simulink model "Target_Control_System"  (R2021b)
settings: Solver=FixedStepDiscrete  StartTime=0.0  StopTime=5  RelTol=1e-3
PreLoadFcn:
  | RTWConfigurationCB('preloadfcn', bdroot);
PostLoadFcn:
  | load('configuration/data_struct.mat');
  | load('configuration/fluxMaps_propMotor.mat');
  | load('configuration/parameterInit_PROP.mat');
  | load('configuration/parameterInit_PUMP.mat');
  | load('configuration/parameterInit_PITCH.mat');
  | load('configuration/parameterInit_TILT.mat');
  | %load('configuration/base_workspace_signal_definition.mat');
  | %load('resolvedatastores_to_baseworkspace_for_faster_simulation.mat');
model workspace (MAT data in the model file):
  SIMULATION_OPTIONS : Simulink.Parameter (value not decoded)
  TARGET_CODE_GEN : Simulink.Parameter (value not decoded)
  TCS_SAMPLE_FREQ_HZ : Simulink.Parameter (value not decoded)
symbols that are objects in the model workspace (value not decoded): TARGET_CODE_GEN, TCS_SAMPLE_FREQ_HZ
undefined symbols (not defined in the file): A_DQ_REF_LPF_INIT__PITCH, A_DQ_REF_LPF_INIT__PROP, A_DQ_REF_LPF_INIT__PUMP, A_DQ_REF_LPF_INIT__TILT, A_OBSERVER_CONFIDENCE_INIT__PITCH, A_OBSERVER_CONFIDENCE_INIT__PROP, A_OBSERVER_CONFIDENCE_INIT__PUMP, A_OBSERVER_CONFIDENCE_INIT__TILT, ACTUATOR_MAX_ANGLE_TRIP__PITCH, ACTUATOR_MIN_ANGLE_TRIP__PITCH, ACTUATOR_POS_SENSOR_INV_DIRECTION__PITCH, ACTUATOR_POS_SENSOR_INV_DIRECTION__TILT, ACTUATOR_POS_SENSOR_OFFSET__PITCH, ACTUATOR_POS_SENSOR_OFFSET__TILT, ADC_scaler1_baseaddr_TILT, ADC_SCALER_FLOAT_TO_FIXPOINT_EXPANSION, ANGLE_ELEC_FROM_SENSOR_OFFSET_INIT__PITCH, ANGLE_ELEC_FROM_SENSOR_OFFSET_INIT__PROP, ANGLE_ELEC_FROM_SENSOR_OFFSET_INIT__PUMP, ANGLE_ELEC_FROM_SENSOR_OFFSET_INIT__TILT, AUTO_CLEAR_FAULTS_ENABLED__PITCH, AUTO_CLEAR_FAULTS_ENABLED__PROP, AUTO_CLEAR_FAULTS_ENABLED__PUMP, AUTO_CLEAR_FAULTS_ENABLED__TILT, AUTO_CLEAR_FAULTS_WAIT_TICKS__PITCH, AUTO_CLEAR_FAULTS_WAIT_TICKS__PROP, AUTO_CLEAR_FAULTS_WAIT_TICKS__PUMP, AUTO_CLEAR_FAULTS_WAIT_TICKS__TILT, AUTO_I_ZERO_IDLE_TICKS__PITCH, AUTO_I_ZERO_IDLE_TICKS__PROP, AUTO_I_ZERO_IDLE_TICKS__PUMP, AUTO_I_ZERO_IDLE_TICKS__TILT, AUTO_I_ZERO_OFFSET_IDC_THRESHOLD__PITCH, AUTO_I_ZERO_OFFSET_IDC_THRESHOLD__PROP, AUTO_I_ZERO_OFFSET_IDC_THRESHOLD__PUMP, AUTO_I_ZERO_OFFSET_IDC_THRESHOLD__TILT, AUTO_I_ZERO_OFFSET_IPH_THRESHOLD__PITCH, AUTO_I_ZERO_OFFSET_IPH_THRESHOLD__PROP, AUTO_I_ZERO_OFFSET_IPH_THRESHOLD__PUMP, AUTO_I_ZERO_OFFSET_IPH_THRESHOLD__TILT, AUTO_SENSORLESS_SWITCHOVER_DISABLE_OMEGA, AUTO_SENSORLESS_SWITCHOVER_ENABLE_OMEGA, AUTO_SENSORLESS_SWITCHOVER_MIN_CONFIDENCE, AUXILIARY_PROTECTION_UNIT_BASEADDR__TILT, blanking_max_error_omega_INIT_PITCH, blanking_max_error_omega_INIT_TILT, blanking_max_error_position_INIT_PITCH, blanking_max_error_position_INIT_TILT, BRUTE_START_I_Q_REF_RAMP_SPEED__PITCH, BRUTE_START_I_Q_REF_RAMP_SPEED__PROP, BRUTE_START_I_Q_REF_RAMP_SPEED__PUMP, BRUTE_START_I_Q_REF_RAMP_SPEED__TILT, CONTROL_LOOP_DT_INIT__PITCH, CONTROL_LOOP_DT_INIT__PROP, CONTROL_LOOP_DT_INIT__PUMP, CONTROL_LOOP_DT_INIT__TILT, CORRECTION_FILTER_SCALE__PITCH, CORRECTION_FILTER_SCALE__PROP, CORRECTION_FILTER_SCALE__PUMP, CORRECTION_FILTER_SCALE__TILT ... (+458)
libraries: simulink x178, Reusables_Lib x24
(part 35 of 47)

== system Target_Control_System/Target_Control_System/MainLoop/tiltMotor_mainLoop/mainTask_tilt/motorTaskMainFastStep(&oTilt)/Control Loops - Tilt/Position Controller Tilt ==
  oRampDataPos_.fRampOut : Inport
  Enable : EnablePort
  Connect PosController to CurrentController : Subsystem
  Data Store Read1 : DataStoreRead  DataStoreName=oTilt  DataStoreElements=oTilt.oMot_.oParam_.fPosition2currentPMultiplier_  IndexOptions=Index vector (dialog)  Indices=1  OutputSizes=1
  Data Store Read10 : DataStoreRead  DataStoreName=oTilt  DataStoreElements=oTilt.oMot_.oState_.oPosSensor_.oPidDataPosCtrl_.oParameter_.ipInhibitTarget_  IndexOptions=Index vector (dialog)  Indices=1  OutputSizes=1
  Data Store Read11 : DataStoreRead  DataStoreName=oTilt  DataStoreElements=oTilt.oMot_.oState_.oPosSensor_.oPidDataPosCtrl_.oParameter_.fLoopDt_  IndexOptions=Index vector (dialog)  Indices=1  OutputSizes=1
  Data Store Read12 : DataStoreRead  DataStoreName=oTilt  DataStoreElements=oTilt.oMot_.oState_.oPosSensor_.oPidDataPosCtrl_.oParameter_.fIntMax_  IndexOptions=Index vector (dialog)  Indices=1  OutputSizes=1
  Data Store Read13 : DataStoreRead  DataStoreName=oTilt  DataStoreElements=oTilt.oMot_.oState_.oPosSensor_.oPidDataPosCtrl_.oParameter_.fIntMin_  IndexOptions=Index vector (dialog)  Indices=1  OutputSizes=1
  Data Store Read14 : DataStoreRead  DataStoreName=oTilt  DataStoreElements=oTilt.oMot_.oState_.oPosSensor_.oPidDataPosCtrl_.oParameter_.fIntegratorLeakFactor_  IndexOptions=Index vector (dialog)  Indices=1  OutputSizes=1
  Data Store Read15 : DataStoreRead  DataStoreName=oTilt  DataStoreElements=oTilt.oMot_.oState_.oPosSensor_.oPidDataPosCtrl_.oParameter_.fKd_  IndexOptions=Index vector (dialog)  Indices=1  OutputSizes=1
  Data Store Read16 : DataStoreRead  DataStoreName=oTilt  DataStoreElements=oTilt.oMot_.oState_.oPosSensor_.fOmegaEFromSensor_  IndexOptions=Index vector (dialog)  Indices=1  OutputSizes=1
  Data Store Read17 : DataStoreRead  DataStoreName=oTilt  DataStoreElements=oTilt.oMot_.oState_.oPosSensor_.oPidDataPosCtrl_.oParameter_.fDMax_  IndexOptions=Index vector (dialog)  Indices=1  OutputSizes=1
  Data Store Read18 : DataStoreRead  DataStoreName=oTilt  DataStoreElements=oTilt.oMot_.oState_.oPosSensor_.oPidDataPosCtrl_.oParameter_.fDMin_  IndexOptions=Index vector (dialog)  Indices=1  OutputSizes=1
  Data Store Read19 : DataStoreRead  DataStoreName=oTilt  DataStoreElements=oTilt.oMot_.oState_.oPosSensor_.oPidDataPosCtrl_.oParameter_.fKp_  IndexOptions=Index vector (dialog)  Indices=1  OutputSizes=1
  Data Store Read2 : DataStoreRead  DataStoreName=oTilt  DataStoreElements=oTilt.oMot_.oParam_.fPosition2currentIMultiplier_  IndexOptions=Index vector (dialog)  Indices=1  OutputSizes=1
  Data Store Read20 : DataStoreRead  DataStoreName=oTilt  DataStoreElements=oTilt.oMot_.oState_.oPosSensor_.oPidDataPosCtrl_.oParameter_.fOutMax_  IndexOptions=Index vector (dialog)  Indices=1  OutputSizes=1
  Data Store Read21 : DataStoreRead  DataStoreName=oTilt  DataStoreElements=oTilt.oMot_.oState_.oPosSensor_.oPidDataPosCtrl_.oParameter_.fOutMin_  IndexOptions=Index vector (dialog)  Indices=1  OutputSizes=1
  Data Store Read22 : DataStoreRead  DataStoreName=oTilt  DataStoreElements=oTilt.oMot_.oState_.oPosSensor_.oPidDataPosCtrl_.fState_  IndexOptions=Index vector (dialog)  Indices=1  OutputSizes=1
  Data Store Read3 : DataStoreRead  DataStoreName=oTilt  DataStoreElements=oTilt.oMot_.oState_.oPosSensor_.oGbx_.fCurrentOutputAngle_  IndexOptions=Index vector (dialog)  Indices=1  OutputSizes=1
  Data Store Read4 : DataStoreRead  DataStoreName=oTilt  DataStoreElements=oTilt.oMot_.oParam_.fPosition2currentDMultiplier_  IndexOptions=Index vector (dialog)  Indices=1  OutputSizes=1
  Data Store Read5 : DataStoreRead  DataStoreName=oTilt  DataStoreElements=oTilt.oMot_.oState_.oPosSensor_.oPidDataPosCtrl_.oParameter_.fErrorReduction_  IndexOptions=Index vector (dialog)  Indices=1  OutputSizes=1
  Data Store Read6 : DataStoreRead  DataStoreName=oTilt  DataStoreElements=oTilt.oMot_.oState_.oPosSensor_.oPidDataPosCtrl_.oParameter_.fLargeErrorThresholdPositive_  IndexOptions=Index vector (dialog)  Indices=1  OutputSizes=1
  Data Store Read7 : DataStoreRead  DataStoreName=oTilt  DataStoreElements=oTilt.oMot_.oState_.oPosSensor_.oPidDataPosCtrl_.oParameter_.fLargeErrorThresholdNegative_  IndexOptions=Index vector (dialog)  Indices=1  OutputSizes=1
  Data Store Read8 : DataStoreRead  DataStoreName=oTilt  DataStoreElements=oTilt.oMot_.oState_.oPosSensor_.oPidDataPosCtrl_.oParameter_.fBlankingMaxError_  IndexOptions=Index vector (dialog)  Indices=1  OutputSizes=1
  Data Store Read9 : DataStoreRead  DataStoreName=oTilt  DataStoreElements=oTilt.oMot_.oState_.oPosSensor_.oPidDataPosCtrl_.oParameter_.fKi_  IndexOptions=Index vector (dialog)  Indices=1  OutputSizes=1
  Data Store Write : DataStoreWrite  DataStoreName=oTilt  DataStoreElements=oTilt.oMot_.oState_.oPosSensor_.oPidDataPosCtrl_.oParameter_.iLargeErrorPresent_  IndexOptions=Index vector (dialog)  Indices=1  OutputSizes=1
  Data Store Write1 : DataStoreWrite  DataStoreName=oTilt  DataStoreElements=oTilt.oMot_.oState_.oPosSensor_.oPidDataPosCtrl_.oParameter_.fITerm_  IndexOptions=Index vector (dialog)  Indices=1  OutputSizes=1
  Data Store Write2 : DataStoreWrite  DataStoreName=oTilt  DataStoreElements=oTilt.oMot_.oState_.oPosSensor_.oPidDataPosCtrl_.oParameter_.fDTerm_  IndexOptions=Index vector (dialog)  Indices=1  OutputSizes=1
  Data Store Write3 : DataStoreWrite  DataStoreName=oTilt  DataStoreElements=oTilt.oMot_.oState_.oPosSensor_.oPidDataPosCtrl_.oParameter_.fPTerm_  IndexOptions=Index vector (dialog)  Indices=1  OutputSizes=1
  Data Store Write4 : DataStoreWrite  DataStoreName=oTilt  DataStoreElements=oTilt.oMot_.oState_.oRampDataOmegaERef_.fSetpoint_  IndexOptions=Index vector (dialog)  Indices=1  OutputSizes=1
  Data Store Write5 : DataStoreWrite  DataStoreName=oTilt  DataStoreElements=oTilt.oMot_.oState_.oPosSensor_.oPidDataPosCtrl_.fState_  IndexOptions=Index vector (dialog)  Indices=1  OutputSizes=1
  Data Store Write6 : DataStoreWrite  DataStoreName=oTilt  DataStoreElements=oTilt.oMot_.oState_.fIqRefFromSpeedController_  IndexOptions=Index vector (dialog)  Indices=1  OutputSizes=1
  pid2ControllerStep(oPidDataPosCtrl)_pitch : Subsystem  TreatAsAtomicUnit=on
  oRampDataOmegaERef_.fSetpoint : Outport
  wires:
  Data Store Read22/1 -> pid2ControllerStep(oPidDataPosCtrl)_pitch/20(fpState)
  Data Store Read21/1 -> pid2ControllerStep(oPidDataPosCtrl)_pitch/19(fOutMin)
  Data Store Read20/1 -> pid2ControllerStep(oPidDataPosCtrl)_pitch/18(fOutMax)
  Data Store Read19/1 -> pid2ControllerStep(oPidDataPosCtrl)_pitch/17(fKp)
  Data Store Read18/1 -> pid2ControllerStep(oPidDataPosCtrl)_pitch/16(fDMin)
  Data Store Read17/1 -> pid2ControllerStep(oPidDataPosCtrl)_pitch/15(fDMax)
  Data Store Read16/1 -> pid2ControllerStep(oPidDataPosCtrl)_pitch/14(fActualDt)
  Data Store Read15/1 -> pid2ControllerStep(oPidDataPosCtrl)_pitch/13(fKd)
  Data Store Read14/1 -> pid2ControllerStep(oPidDataPosCtrl)_pitch/12(fIntegratorLeakFactor)
  Data Store Read13/1 -> pid2ControllerStep(oPidDataPosCtrl)_pitch/11(fIntMin)
  Data Store Read12/1 -> pid2ControllerStep(oPidDataPosCtrl)_pitch/10(fIntMax)
  Data Store Read11/1 -> pid2ControllerStep(oPidDataPosCtrl)_pitch/9(fLoopDt)
  Data Store Read10/1 -> pid2ControllerStep(oPidDataPosCtrl)_pitch/8(ipInhibitTarget)
  Data Store Read9/1 -> pid2ControllerStep(oPidDataPosCtrl)_pitch/7(fKi)
  Data Store Read8/1 -> pid2ControllerStep(oPidDataPosCtrl)_pitch/6(fBlankingMaxError)
  Data Store Read7/1 -> pid2ControllerStep(oPidDataPosCtrl)_pitch/5(fLargeErrorThresholdNegative)
  Data Store Read6/1 -> pid2ControllerStep(oPidDataPosCtrl)_pitch/4(fLargeErrorThresholdPositive)
  Data Store Read5/1 -> pid2ControllerStep(oPidDataPosCtrl)_pitch/3(fErrorReduction)
  Data Store Read3/1 -> pid2ControllerStep(oPidDataPosCtrl)_pitch/2(fActual)
  oRampDataPos_.fRampOut/1 -> pid2ControllerStep(oPidDataPosCtrl)_pitch/1(fTarget)
  Data Store Read1/1 -> Connect PosController to CurrentController/1(fPMultiplier)
  Data Store Read2/1 -> Connect PosController to CurrentController/2(fIMultiplier)
  Connect PosController to CurrentController/1(fIqRefFromSpeedController) -> Data Store Write6/1
  Data Store Read4/1 -> Connect PosController to CurrentController/3(DMultiplier)
  pid2ControllerStep(oPidDataPosCtrl)_pitch/2(fITerm) -> Connect PosController to CurrentController/4(fITerm), Data Store Write1/1
  pid2ControllerStep(oPidDataPosCtrl)_pitch/4(fPTerm) -> Connect PosController to CurrentController/6(fPTerm), Data Store Write3/1
  pid2ControllerStep(oPidDataPosCtrl)_pitch/3(fDTerm) -> Data Store Write2/1, Connect PosController to CurrentController/5(fDTerm)
  pid2ControllerStep(oPidDataPosCtrl)_pitch/1(iLargeErrorPresent) -> Data Store Write/1
  pid2ControllerStep(oPidDataPosCtrl)_pitch/5(fOutput) -> Data Store Write4/1, oRampDataOmegaERef_.fSetpoint/1
  pid2ControllerStep(oPidDataPosCtrl)_pitch/6(*fpState) -> Data Store Write5/1

== system Target_Control_System/Target_Control_System/MainLoop/tiltMotor_mainLoop/mainTask_tilt/motorTaskMainFastStep(&oTilt)/Control Loops - Tilt/Ramp Flux Feedforward ==
  Enable : EnablePort
  Data Store Read105 : DataStoreRead  DataStoreName=oTilt  DataStoreElements=oTilt.oMot_.oState_.oRampDataFluxFeedforwardGain_.oParam_.fTimestepS_  IndexOptions=Index vector (dialog)  Indices=1  OutputSizes=1
  Data Store Read106 : DataStoreRead  DataStoreName=oTilt  DataStoreElements=oTilt.oMot_.oState_.oRampDataFluxFeedforwardGain_.oParam_.fUpslope_  IndexOptions=Index vector (dialog)  Indices=1  OutputSizes=1
  Data Store Read107 : DataStoreRead  DataStoreName=oTilt  DataStoreElements=oTilt.oMot_.oState_.oRampDataFluxFeedforwardGain_.oParam_.fDownslope_  IndexOptions=Index vector (dialog)  Indices=1  OutputSizes=1
  Data Store Read108 : DataStoreRead  DataStoreName=oTilt  DataStoreElements=oTilt.oMot_.oState_.oRampDataFluxFeedforwardGain_.fSetpoint_  IndexOptions=Index vector (dialog)  Indices=1  OutputSizes=1
  Data Store Write63 : DataStoreWrite  DataStoreName=oTilt  DataStoreElements=oTilt.oMot_.oState_.oRampDataFluxFeedforwardGain_.fRampOutDdt_  IndexOptions=Index vector (dialog)  Indices=1  OutputSizes=1
  Data Store Write66 : DataStoreWrite  DataStoreName=oTilt  DataStoreElements=oTilt.oMot_.oState_.oRampDataFluxFeedforwardGain_.fRampOut_  IndexOptions=Index vector (dialog)  Indices=1  OutputSizes=1
  rampStep(oRampDataFluxFeedforwardGain)_tilt : Reusables_Lib/rampStep_  SystemSampleTime=-1  VariantActivationTime=update diagram  Latency=0  AutoFrameSizeCalculation=off
  wires:
  rampStep(oRampDataFluxFeedforwardGain)_tilt/2 -> Data Store Write63/1
  rampStep(oRampDataFluxFeedforwardGain)_tilt/1 -> Data Store Write66/1
  Data Store Read108/1 -> rampStep(oRampDataFluxFeedforwardGain)_tilt/1
  Data Store Read106/1 -> rampStep(oRampDataFluxFeedforwardGain)_tilt/2
  Data Store Read107/1 -> rampStep(oRampDataFluxFeedforwardGain)_tilt/3
  Data Store Read105/1 -> rampStep(oRampDataFluxFeedforwardGain)_tilt/4

== system Target_Control_System/Target_Control_System/MainLoop/tiltMotor_mainLoop/mainTask_tilt/motorTaskMainFastStep(&oTilt)/Control Loops - Tilt/Speed Controller Tilt ==
  oRampDataOmegaERef_.fRampOut : Inport
  Enable : EnablePort
  AND : Logic  AllPortsSameDT=off  OutDataTypeStr=boolean
  Constant : Constant  Value=245  OutDataTypeStr=int32  SampleTime=-1
  Constant1 : Constant  Value=0  OutDataTypeStr=int32  SampleTime=-1
  Data Store Read1 : DataStoreRead  DataStoreName=oTilt  DataStoreElements=oTilt.oMot_.oParam_.uiTorqueMirroringActive_  IndexOptions=Index vector (dialog)  Indices=1  OutputSizes=1
  Data Store Read2 : DataStoreRead  DataStoreName=oTilt  DataStoreElements=oTilt.oMot_.oState_.uiDriveState_  IndexOptions=Index vector (dialog)  Indices=1  OutputSizes=1
  Data Store Read3 : DataStoreRead  DataStoreName=oTilt  DataStoreElements=oTilt.oIsr_.oParam_.iUseSensorAngle_  IndexOptions=Index vector (dialog)  Indices=1  OutputSizes=1
  GreaterThan : RelationalOperator  Operator=>  OutDataTypeStr=boolean  RndMeth=Simplest
  Less Than : RelationalOperator  Operator=<  OutDataTypeStr=boolean  RndMeth=Simplest
  NOT : Logic  Operator=NOT  IconShape=distinctive  AllPortsSameDT=off  OutDataTypeStr=boolean
  NOT1 : Logic  Operator=NOT  AllPortsSameDT=off  OutDataTypeStr=boolean
  PID2controller_sensoredDrives : Subsystem  TreatAsAtomicUnit=on
  PIcontroller_sensorlessDrives : Subsystem  TreatAsAtomicUnit=on
  Set Iq Ref Tilt : Subsystem  TreatAsAtomicUnit=on
  Switch : Switch  Criteria=u2 > Threshold
  wires:
  PIcontroller_sensorlessDrives/1(fIqRefFromSpeedController) -> Switch/3
  GreaterThan/1 -> PID2controller_sensoredDrives/Enable, Switch/2, NOT1/1
  Constant1/1 -> GreaterThan/2
  Data Store Read3/1 -> GreaterThan/1
  NOT1/1 -> PIcontroller_sensorlessDrives/Enable
  PID2controller_sensoredDrives/1(fIqRefFromSpeedController) -> Switch/1
  Switch/1 -> Set Iq Ref Tilt/1(fIqRefFromSpeedController)
  oRampDataOmegaERef_.fRampOut/1 -> PID2controller_sensoredDrives/1(oRampDataOmegaERef_.fRampOut), PIcontroller_sensorlessDrives/1(oRampDataOmegaERef_.fRampOut)
  Data Store Read2/1 -> Less Than/1
  Data Store Read1/1 -> NOT/1
  Constant/1 -> Less Than/2
  NOT/1 -> AND/1
  Less Than/1 -> AND/2
  AND/1 -> Set Iq Ref Tilt/Enable

== system Target_Control_System/Target_Control_System/MainLoop/tiltMotor_mainLoop/mainTask_tilt/motorTaskMainFastStep(&oTilt)/Correction Constants for Observer and Control - Tilt/1//sqrt(1+u^2)1 ==
  fTemp : Inport
  Add : Sum
  Constant2 : Constant  OutDataTypeStr=single
  Constant3 : Constant  OutDataTypeStr=single
  Divide5 : Product  Inputs=**
  Divide6 : Product  Inputs=*/
  Sqrt : Sqrt  SaturateOnIntegerOverflow=on
  Out1 : Outport
  wires:
  Divide5/1 -> Add/1
  fTemp/1 -> Divide5/1, Divide5/2
  Add/1 -> Sqrt/1
  Sqrt/1 -> Divide6/2
  Constant3/1 -> Divide6/1
  Constant2/1 -> Add/2
  Divide6/1 -> Out1/1

== system Target_Control_System/Target_Control_System/MainLoop/tiltMotor_mainLoop/mainTask_tilt/motorTaskMainFastStep(&oTilt)/Mechanical System - Tilt/processSensors(&oPitch) ==
  Enable : EnablePort
  Auxiliary sensor : Subsystem
  Data Store Read94 : DataStoreRead  DataStoreName=oTilt  DataStoreElements=oTilt.oMot_.oState_.oPosSensor_.eAuxiliaryPositionSensorType_  IndexOptions=Index vector (dialog)  Indices=1  OutputSizes=1
  Enumerated Constant2 : simulink/Sources/Enumerated Constant  OutDataTypeStr=Enum: EPositionSensor_t  Value=EPositionSensor_t.eNone  SampleTime=-1
  Input (motor) side sensor : Subsystem
  NotEqual : RelationalOperator  Operator=~=  OutDataTypeStr=boolean  RndMeth=Simplest
  Output (actuator) side sensor : Subsystem
  wires:
  NotEqual/1 -> Auxiliary sensor/Enable
  Enumerated Constant2/1 -> NotEqual/2
  Data Store Read94/1 -> NotEqual/1

== system Target_Control_System/Target_Control_System/MainLoop/tiltMotor_mainLoop/mainTask_tilt/motorTaskMainFastStep(&oTilt)/Motor Acceleration - Tilt/First filter stage ==
  function : TriggerPort  TriggerType=function-call  VariantControl=Variant
  Data Store Read : DataStoreRead  DataStoreName=mdl_tilt_fOmegaE  IndexOptions=Index vector (dialog)  Indices=1  OutputSizes=1
  Data Store Read1 : DataStoreRead  DataStoreName=oTilt  DataStoreElements=oTilt.oMot_.oState_.oMotorAccelerationFilterStage1_.afConstantsA_.h0  IndexOptions=Index vector (dialog)  Indices=1  OutputSizes=1
  Data Store Read10 : DataStoreRead  DataStoreName=oTilt  DataStoreElements=oTilt.oMot_.oState_.oMotorAccelerationFilterStage1_.afPreviousOutputs_.h1  IndexOptions=Index vector (dialog)  Indices=1  OutputSizes=1
  Data Store Read11 : DataStoreRead  DataStoreName=oTilt  DataStoreElements=oTilt.oMot_.oState_.fOmegaEPrevious_  IndexOptions=Index vector (dialog)  Indices=1  OutputSizes=1
  Data Store Read2 : DataStoreRead  DataStoreName=oTilt  DataStoreElements=oTilt.oMot_.oState_.oMotorAccelerationFilterStage1_.afConstantsA_.h1  IndexOptions=Index vector (dialog)  Indices=1  OutputSizes=1
  Data Store Read3 : DataStoreRead  DataStoreName=oTilt  DataStoreElements=oTilt.oMot_.oState_.oMotorAccelerationFilterStage1_.afConstantsA_.h2  IndexOptions=Index vector (dialog)  Indices=1  OutputSizes=1
  Data Store Read4 : DataStoreRead  DataStoreName=oTilt  DataStoreElements=oTilt.oMot_.oState_.oMotorAccelerationFilterStage1_.afConstantsB_.h0  IndexOptions=Index vector (dialog)  Indices=1  OutputSizes=1
  Data Store Read5 : DataStoreRead  DataStoreName=oTilt  DataStoreElements=oTilt.oMot_.oState_.oMotorAccelerationFilterStage1_.afConstantsB_.h1  IndexOptions=Index vector (dialog)  Indices=1  OutputSizes=1
  Data Store Read6 : DataStoreRead  DataStoreName=oTilt  DataStoreElements=oTilt.oMot_.oState_.oMotorAccelerationFilterStage1_.afConstantsB_.h2  IndexOptions=Index vector (dialog)  Indices=1  OutputSizes=1
  Data Store Read7 : DataStoreRead  DataStoreName=oTilt  DataStoreElements=oTilt.oMot_.oState_.oMotorAccelerationFilterStage1_.afPreviousInputs_.h0  IndexOptions=Index vector (dialog)  Indices=1  OutputSizes=1
  Data Store Read8 : DataStoreRead  DataStoreName=oTilt  DataStoreElements=oTilt.oMot_.oState_.oMotorAccelerationFilterStage1_.afPreviousInputs_.h1  IndexOptions=Index vector (dialog)  Indices=1  OutputSizes=1
  Data Store Read9 : DataStoreRead  DataStoreName=oTilt  DataStoreElements=oTilt.oMot_.oState_.oMotorAccelerationFilterStage1_.afPreviousOutputs_.h0  IndexOptions=Index vector (dialog)  Indices=1  OutputSizes=1
  Data Store Write1 : DataStoreWrite  DataStoreName=oTilt  DataStoreElements=oTilt.oMot_.oState_.oMotorAccelerationFilterStage1_.fFilterOutput_  IndexOptions=Index vector (dialog)  Indices=1  OutputSizes=1
  Data Store Write2 : DataStoreWrite  DataStoreName=oTilt  DataStoreElements=oTilt.oMot_.oState_.oMotorAccelerationFilterStage1_.afPreviousOutputs_.h0  IndexOptions=Index vector (dialog)  Indices=1  OutputSizes=1
  Data Store Write3 : DataStoreWrite  DataStoreName=oTilt  DataStoreElements=oTilt.oMot_.oState_.oMotorAccelerationFilterStage1_.afPreviousOutputs_.h1  IndexOptions=Index vector (dialog)  Indices=1  OutputSizes=1
  Data Store Write4 : DataStoreWrite  DataStoreName=oTilt  DataStoreElements=oTilt.oMot_.oState_.oMotorAccelerationFilterStage1_.afPreviousInputs_.h0  IndexOptions=Index vector (dialog)  Indices=1  OutputSizes=1
  Data Store Write5 : DataStoreWrite  DataStoreName=oTilt  DataStoreElements=oTilt.oMot_.oState_.oMotorAccelerationFilterStage1_.afPreviousInputs_.h1  IndexOptions=Index vector (dialog)  Indices=1  OutputSizes=1
  Subtract : Sum  Inputs=+-
  softwareIirFilterStep() : Subsystem
  wires:
  softwareIirFilterStep()/3(*afPreviousOutputs1) -> Data Store Write3/1
  Data Store Read3/1 -> softwareIirFilterStep()/7(afConstantsA2)
  Data Store Read11/1 -> Subtract/2
  Subtract/1 -> softwareIirFilterStep()/1(newInput)
  softwareIirFilterStep()/5(fFilterOutput) -> Data Store Write1/1
  Data Store Read6/1 -> softwareIirFilterStep()/4(afConstantsB2)
  Data Store Read8/1 -> softwareIirFilterStep()/9(afPreviousInputs1)
  Data Store Read/1 -> Subtract/1
  Data Store Read7/1 -> softwareIirFilterStep()/8(afPreviousInputs0)
  Data Store Read1/1 -> softwareIirFilterStep()/5(afConstantsA0)
  Data Store Read10/1 -> softwareIirFilterStep()/11(afPreviousOutputs1)
  softwareIirFilterStep()/1(*afPreviousInputs1) -> Data Store Write5/1
  softwareIirFilterStep()/4(*afPreviousOutputs0) -> Data Store Write2/1
  softwareIirFilterStep()/2(*afPreviousInputs0) -> Data Store Write4/1
  Data Store Read2/1 -> softwareIirFilterStep()/6(afConstantsA1)
  Data Store Read9/1 -> softwareIirFilterStep()/10(afPreviousOutputs0)
  Data Store Read5/1 -> softwareIirFilterStep()/3(afConstantsB1)
  Data Store Read4/1 -> softwareIirFilterStep()/2(afConstantsB0)

== system Target_Control_System/Target_Control_System/MainLoop/tiltMotor_mainLoop/mainTask_tilt/motorTaskMainFastStep(&oTilt)/Motor Acceleration - Tilt/Speed step ==
  function : TriggerPort  TriggerType=function-call  VariantControl=Variant
  Data Store Read : DataStoreRead  DataStoreName=mdl_tilt_fOmegaE  IndexOptions=Index vector (dialog)  Indices=1  OutputSizes=1
  Data Store Write : DataStoreWrite  DataStoreName=oTilt  DataStoreElements=oTilt.oMot_.oState_.fOmegaEPrevious_  IndexOptions=Index vector (dialog)  Indices=1  OutputSizes=1
  wires:
  Data Store Read/1 -> Data Store Write/1

== system Target_Control_System/Target_Control_System/MainLoop/tiltMotor_mainLoop/mainTask_tilt/motorTaskMainFastStep(&oTilt)/Observer Confidence - Tilt/IIR1 ==
  In : Inport
  1-K : Inport  Port=2
  K : Inport  Port=3
  Product : Product  OutDataTypeStr=single  RndMeth=Zero
  Product1 : Product  RndMeth=Zero
  Sum : Sum  Inputs=|++  OutDataTypeStr=single
  Unit Delay : UnitDelay  SampleTime=-1  HasFrameUpgradeWarning=on
  Out : Outport
  wires:
  Sum/1 -> Unit Delay/1, Out/1
  Unit Delay/1 -> Product/1
  K/1 -> Product1/2
  1-K/1 -> Product/2
  Product/1 -> Sum/1
  Product1/1 -> Sum/2
  In/1 -> Product1/1

== system Target_Control_System/Target_Control_System/MainLoop/tiltMotor_mainLoop/mainTask_tilt/motorTaskMainFastStep(&oTilt)/Software Overcurrent Protection - Tilt/Forced_angle_overcurrent ==
  Enable : EnablePort
  Chart : Stateflow chart  TreatAsAtomicUnit=on

== system Target_Control_System/Target_Control_System/MainLoop/tiltMotor_mainLoop/mainTask_tilt/motorTaskMainFastStep(&oTilt)/Software Overcurrent Protection - Tilt/checkForHwOvercurrents(&oTilt) ==
  Enable : EnablePort
  "checkForHwOvercurrents " : Stateflow chart  TreatAsAtomicUnit=on
  gateDriverStatus : Subsystem  Variant=on

== system Target_Control_System/Target_Control_System/Simulation Controls/Simulation Data Store Initialization/parameter_init_prop/initializeMotorTaskParameterPropulsion()/Sim Options Prop Forced Angle Variant Subsystem/Sim Options 0 Prop Forced Angle Subsystem ==
  Constant59 : Constant  Value=FORCED_ANGLE_START_INIT__PROP  OutDataTypeStr=uint32  SampleTime=-1
  Out1 : Outport
  wires:
  Constant59/1 -> Out1/1

== system Target_Control_System/Target_Control_System/Simulation Controls/Simulation Data Store Initialization/parameter_init_prop/initializeMotorTaskParameterPropulsion()/Sim Options Prop Forced Angle Variant Subsystem/Sim Options 1 Prop Forced Angle Subsystem ==
  Constant : Constant  Value=0  OutDataTypeStr=uint32
  Out1 : Outport
  wires:
  Constant/1 -> Out1/1

== system Target_Control_System/Target_Control_System/Simulation Controls/Simulation Data Store Initialization/parameter_init_pump/initializeMotorTaskParameterPump()/Sim Options Pump Forced Angle Variant Subsystem/Sim Options 0 Pump Forced Angle Subsystem ==
  Constant59 : Constant  Value=FORCED_ANGLE_START_INIT__PUMP  OutDataTypeStr=uint32  SampleTime=-1
  Out1 : Outport
  wires:
  Constant59/1 -> Out1/1

== system Target_Control_System/Target_Control_System/Simulation Controls/Simulation Data Store Initialization/parameter_init_pump/initializeMotorTaskParameterPump()/Sim Options Pump Forced Angle Variant Subsystem/Sim Options 1 Pump Forced Angle Subsystem ==
  Constant : Constant  Value=0  OutDataTypeStr=uint32
  Out1 : Outport
  wires:
  Constant/1 -> Out1/1

== system Target_Control_System/Target_Control_System/Simulation Controls/Simulation Data Store Initialization/setTiltMotorSpecificParameters()/Enabled Subsystem MotorType/Switch Case Action Subsystem MotorType12/Switch Case Action Subsystem Motor Type1 ==
  Action Port : ActionPort  ActionPortLabel=case [ 1 ]:
  Constant14 : Constant  Value=POSITION_CONTROL_SETMIN__TILT_WINGTIP  OutDataTypeStr=single
  Constant15 : Constant  Value=POSITION_CONTROL_SETMAX__TILT_WINGTIP  OutDataTypeStr=single
  Constant16 : Constant  Value=GBX_MAX_ANGLE_TRIP__TILT_WINGTIP  OutDataTypeStr=single
  Constant17 : Constant  Value=GBX_MIN_ANGLE_TRIP__TILT_WINGTIP  OutDataTypeStr=single
  Data Store Write15 : DataStoreWrite  DataStoreName=oTilt  DataStoreElements=oTilt.oMot_.oParam_.fPositionSetpointMin_  IndexOptions=Index vector (dialog)  Indices=1  OutputSizes=1
  Data Store Write16 : DataStoreWrite  DataStoreName=oTilt  DataStoreElements=oTilt.oMot_.oParam_.fPositionSetpointMax_  IndexOptions=Index vector (dialog)  Indices=1  OutputSizes=1
  Data Store Write17 : DataStoreWrite  Commented=on  DataStoreName=oTilt  DataStoreElements=oTilt.oMot_.oState_.oPosSensor_.fGbxAngleMaxTrip_  IndexOptions=Index vector (dialog)  Indices=1  OutputSizes=1
  Data Store Write18 : DataStoreWrite  Commented=on  DataStoreName=oTilt  DataStoreElements=oTilt.oMot_.oState_.oPosSensor_.fGbxAngleMinTrip_  IndexOptions=Index vector (dialog)  Indices=1  OutputSizes=1
  maxTrip : Outport
  minTrip : Outport  Port=2
  wires:
  Constant16/1 -> maxTrip/1, Data Store Write17/1
  Constant17/1 -> minTrip/1, Data Store Write18/1
  Constant14/1 -> Data Store Write15/1
  Constant15/1 -> Data Store Write16/1

== system Target_Control_System/Target_Control_System/Simulation Controls/Simulation Data Store Initialization/setTiltMotorSpecificParameters()/Enabled Subsystem MotorType/Switch Case Action Subsystem MotorType12/Switch Case Action Subsystem Motor Type2 ==
  Action Port : ActionPort  ActionPortLabel=case [ 2 ]:
  Constant14 : Constant  Value=POSITION_CONTROL_SETMIN__TILT_TAILTIP  OutDataTypeStr=single
  Constant15 : Constant  Value=POSITION_CONTROL_SETMAX__TILT_TAILTIP  OutDataTypeStr=single
  Constant16 : Constant  Value=GBX_MAX_ANGLE_TRIP__TILT_TAILTIP  OutDataTypeStr=single
  Constant17 : Constant  Value=GBX_MIN_ANGLE_TRIP__TILT_TAILTIP  OutDataTypeStr=single
  Data Store Write15 : DataStoreWrite  DataStoreName=oTilt  DataStoreElements=oTilt.oMot_.oParam_.fPositionSetpointMin_  IndexOptions=Index vector (dialog)  Indices=1  OutputSizes=1
  Data Store Write16 : DataStoreWrite  DataStoreName=oTilt  DataStoreElements=oTilt.oMot_.oParam_.fPositionSetpointMax_  IndexOptions=Index vector (dialog)  Indices=1  OutputSizes=1
  Data Store Write17 : DataStoreWrite  Commented=on  DataStoreName=oTilt  DataStoreElements=oTilt.oMot_.oState_.oPosSensor_.fGbxAngleMaxTrip_  IndexOptions=Index vector (dialog)  Indices=1  OutputSizes=1
  Data Store Write18 : DataStoreWrite  Commented=on  DataStoreName=oTilt  DataStoreElements=oTilt.oMot_.oState_.oPosSensor_.fGbxAngleMinTrip_  IndexOptions=Index vector (dialog)  Indices=1  OutputSizes=1
  maxTrip : Outport
  minTrip : Outport  Port=2
  wires:
  Constant17/1 -> minTrip/1, Data Store Write18/1
  Constant16/1 -> maxTrip/1, Data Store Write17/1
  Constant15/1 -> Data Store Write16/1
  Constant14/1 -> Data Store Write15/1

== system Target_Control_System/Target_Control_System/Simulation Controls/Simulation Data Store Initialization/setTiltMotorSpecificParameters()/Enabled Subsystem MotorType/Switch Case Action Subsystem MotorType3/softwareIirFilterInitialize() ==
  fFreq3db : Inport  OutDataTypeStr=single
  fFreqSample : Inport  Port=2  OutDataTypeStr=single
  Constant : Constant  OutDataTypeStr=single
  Constant1 : Constant  Value=0  OutDataTypeStr=single
  Data Store Write : DataStoreWrite  DataStoreName=oTilt  DataStoreElements=oTilt.oMot_.oState_.oFilterDataForSpeedControlIqRef_.afConstantsA_.h0  IndexOptions=Index vector (dialog)  Indices=1  OutputSizes=1
  Data Store Write1 : DataStoreWrite  DataStoreName=oTilt  DataStoreElements=oTilt.oMot_.oState_.oFilterDataForSpeedControlIqRef_.afConstantsA_.h1  IndexOptions=Index vector (dialog)  Indices=1  OutputSizes=1
  Data Store Write10 : DataStoreWrite  DataStoreName=oTilt  DataStoreElements=oTilt.oMot_.oState_.oFilterDataForSpeedControlIqRef_.fFilterOutput_  IndexOptions=Index vector (dialog)  Indices=1  OutputSizes=1
  Data Store Write2 : DataStoreWrite  DataStoreName=oTilt  DataStoreElements=oTilt.oMot_.oState_.oFilterDataForSpeedControlIqRef_.afConstantsA_.h2  IndexOptions=Index vector (dialog)  Indices=1  OutputSizes=1
  Data Store Write3 : DataStoreWrite  DataStoreName=oTilt  DataStoreElements=oTilt.oMot_.oState_.oFilterDataForSpeedControlIqRef_.afConstantsB_.h2  IndexOptions=Index vector (dialog)  Indices=1  OutputSizes=1
  Data Store Write4 : DataStoreWrite  DataStoreName=oTilt  DataStoreElements=oTilt.oMot_.oState_.oFilterDataForSpeedControlIqRef_.afConstantsB_.h1  IndexOptions=Index vector (dialog)  Indices=1  OutputSizes=1
  Data Store Write5 : DataStoreWrite  DataStoreName=oTilt  DataStoreElements=oTilt.oMot_.oState_.oFilterDataForSpeedControlIqRef_.afConstantsB_.h0  IndexOptions=Index vector (dialog)  Indices=1  OutputSizes=1
  Data Store Write6 : DataStoreWrite  DataStoreName=oTilt  DataStoreElements=oTilt.oMot_.oState_.oFilterDataForSpeedControlIqRef_.afPreviousInputs_.h0  IndexOptions=Index vector (dialog)  Indices=1  OutputSizes=1
  Data Store Write7 : DataStoreWrite  DataStoreName=oTilt  DataStoreElements=oTilt.oMot_.oState_.oFilterDataForSpeedControlIqRef_.afPreviousInputs_.h1  IndexOptions=Index vector (dialog)  Indices=1  OutputSizes=1
  Data Store Write8 : DataStoreWrite  DataStoreName=oTilt  DataStoreElements=oTilt.oMot_.oState_.oFilterDataForSpeedControlIqRef_.afPreviousOutputs_.h0  IndexOptions=Index vector (dialog)  Indices=1  OutputSizes=1
  Data Store Write9 : DataStoreWrite  DataStoreName=oTilt  DataStoreElements=oTilt.oMot_.oState_.oFilterDataForSpeedControlIqRef_.afPreviousOutputs_.h1  IndexOptions=Index vector (dialog)  Indices=1  OutputSizes=1
  Data Type Conversion{1..5} (5 alike) : DataTypeConversion  OutDataTypeStr=single
  Demux : Demux  Outputs=6
  Divide : Product  Inputs=*/  OutDataTypeStr=single
  computeCoefficientsButter() : Subsystem
  fActualFrequencyHz : Outport
  wires:
  computeCoefficientsButter()/2(fFreq3db) -> fActualFrequencyHz/1
  fFreq3db/1 -> computeCoefficientsButter()/1(fCutoffFrequencyHz)
  computeCoefficientsButter()/1(dpOutArray) -> Demux/1
  Demux/6 -> Data Type Conversion5/1
  Demux/5 -> Data Type Conversion4/1
  Demux/3 -> Data Type Conversion3/1
  Demux/4 -> Divide/2
  Divide/1 -> Data Store Write/1
  Constant/1 -> Divide/1
  Demux/2 -> Data Type Conversion1/1
  Demux/1 -> Data Type Conversion2/1
  Constant1/1 -> Data Store Write8/1, Data Store Write10/1, Data Store Write9/1, Data Store Write7/1, Data Store Write6/1
  fFreqSample/1 -> computeCoefficientsButter()/2(dSampleFrequencyHz)
  Data Type Conversion2/1 -> Data Store Write5/1
  Data Type Conversion1/1 -> Data Store Write4/1
  Data Type Conversion3/1 -> Data Store Write3/1
  Data Type Conversion4/1 -> Data Store Write1/1
  Data Type Conversion5/1 -> Data Store Write2/1

== system Target_Control_System/Target_Control_System/Simulation Controls/Simulation Data Store Initialization/setupPwm(&oTilt)/setPwmFrequencyApplication()_tilt/setPwmFrequency()_tilt/softwareIirFilterInitialize() ==
  fFreq3db : Inport
  fFreqSample : Inport  Port=2
  Constant : Constant  OutDataTypeStr=single
  Constant1 : Constant  Value=0  OutDataTypeStr=single
  Data Store Write : DataStoreWrite  DataStoreName=oTilt  DataStoreElements=oTilt.oMot_.oState_.oMotorAccelerationFilterStage1_.afConstantsA_.h0  IndexOptions=Index vector (dialog)  Indices=1  OutputSizes=1
  Data Store Write1 : DataStoreWrite  DataStoreName=oTilt  DataStoreElements=oTilt.oMot_.oState_.oMotorAccelerationFilterStage1_.afConstantsA_.h1  IndexOptions=Index vector (dialog)  Indices=1  OutputSizes=1
  Data Store Write10 : DataStoreWrite  DataStoreName=oTilt  DataStoreElements=oTilt.oMot_.oState_.oMotorAccelerationFilterStage1_.fFilterOutput_  IndexOptions=Index vector (dialog)  Indices=1  OutputSizes=1
  Data Store Write2 : DataStoreWrite  DataStoreName=oTilt  DataStoreElements=oTilt.oMot_.oState_.oMotorAccelerationFilterStage1_.afConstantsA_.h2  IndexOptions=Index vector (dialog)  Indices=1  OutputSizes=1
  Data Store Write3 : DataStoreWrite  DataStoreName=oTilt  DataStoreElements=oTilt.oMot_.oState_.oMotorAccelerationFilterStage1_.afConstantsB_.h2  IndexOptions=Index vector (dialog)  Indices=1  OutputSizes=1
  Data Store Write4 : DataStoreWrite  DataStoreName=oTilt  DataStoreElements=oTilt.oMot_.oState_.oMotorAccelerationFilterStage1_.afConstantsB_.h1  IndexOptions=Index vector (dialog)  Indices=1  OutputSizes=1
  Data Store Write5 : DataStoreWrite  DataStoreName=oTilt  DataStoreElements=oTilt.oMot_.oState_.oMotorAccelerationFilterStage1_.afConstantsB_.h0  IndexOptions=Index vector (dialog)  Indices=1  OutputSizes=1
  Data Store Write6 : DataStoreWrite  DataStoreName=oTilt  DataStoreElements=oTilt.oMot_.oState_.oMotorAccelerationFilterStage1_.afPreviousInputs_.h0  IndexOptions=Index vector (dialog)  Indices=1  OutputSizes=1
  Data Store Write7 : DataStoreWrite  DataStoreName=oTilt  DataStoreElements=oTilt.oMot_.oState_.oMotorAccelerationFilterStage1_.afPreviousInputs_.h1  IndexOptions=Index vector (dialog)  Indices=1  OutputSizes=1
  Data Store Write8 : DataStoreWrite  DataStoreName=oTilt  DataStoreElements=oTilt.oMot_.oState_.oMotorAccelerationFilterStage1_.afPreviousOutputs_.h0  IndexOptions=Index vector (dialog)  Indices=1  OutputSizes=1
  Data Store Write9 : DataStoreWrite  DataStoreName=oTilt  DataStoreElements=oTilt.oMot_.oState_.oMotorAccelerationFilterStage1_.afPreviousOutputs_.h1  IndexOptions=Index vector (dialog)  Indices=1  OutputSizes=1
  Data Type Conversion{1..5} (5 alike) : DataTypeConversion  OutDataTypeStr=single
  Demux : Demux  Outputs=6
  Divide : Product  Inputs=*/  OutDataTypeStr=single
  computeCoefficientsButter() : Subsystem
  fActualFrequencyHz : Outport
  wires:
  Data Type Conversion5/1 -> Data Store Write2/1
  Data Type Conversion4/1 -> Data Store Write1/1
  Data Type Conversion3/1 -> Data Store Write3/1
  Data Type Conversion1/1 -> Data Store Write4/1
  Data Type Conversion2/1 -> Data Store Write5/1
  fFreqSample/1 -> computeCoefficientsButter()/2(dSampleFrequencyHz)
  Constant1/1 -> Data Store Write6/1, Data Store Write7/1, Data Store Write9/1, Data Store Write10/1, Data Store Write8/1
  Demux/1 -> Data Type Conversion2/1
  Demux/2 -> Data Type Conversion1/1
  Constant/1 -> Divide/1
  Divide/1 -> Data Store Write/1
  Demux/4 -> Divide/2
  Demux/3 -> Data Type Conversion3/1
  Demux/5 -> Data Type Conversion4/1
  Demux/6 -> Data Type Conversion5/1
  computeCoefficientsButter()/1(dpOutArray) -> Demux/1
  fFreq3db/1 -> computeCoefficientsButter()/1(fCutoffFrequencyHz)
  computeCoefficientsButter()/2(fFreq3db) -> fActualFrequencyHz/1

== system Target_Control_System/Target_Control_System/Simulation Controls/Simulation Data Store Initialization/setupPwm(&oTilt)/setPwmFrequencyApplication()_tilt/setPwmFrequency()_tilt/softwareIirFilterInitialize()1 ==
  fFreq3db : Inport
  fFreqSample : Inport  Port=2
  Constant : Constant  OutDataTypeStr=single
  Constant1 : Constant  Value=0  OutDataTypeStr=single
  Data Store Write : DataStoreWrite  DataStoreName=oTilt  DataStoreElements=oTilt.oMot_.oState_.oFilterDataForSpeedControlIqRef_.afConstantsA_.h0  IndexOptions=Index vector (dialog)  Indices=1  OutputSizes=1
  Data Store Write1 : DataStoreWrite  DataStoreName=oTilt  DataStoreElements=oTilt.oMot_.oState_.oFilterDataForSpeedControlIqRef_.afConstantsA_.h1  IndexOptions=Index vector (dialog)  Indices=1  OutputSizes=1
  Data Store Write10 : DataStoreWrite  DataStoreName=oTilt  DataStoreElements=oTilt.oMot_.oState_.oFilterDataForSpeedControlIqRef_.fFilterOutput_  IndexOptions=Index vector (dialog)  Indices=1  OutputSizes=1
  Data Store Write2 : DataStoreWrite  DataStoreName=oTilt  DataStoreElements=oTilt.oMot_.oState_.oFilterDataForSpeedControlIqRef_.afConstantsA_.h2  IndexOptions=Index vector (dialog)  Indices=1  OutputSizes=1
  Data Store Write3 : DataStoreWrite  DataStoreName=oTilt  DataStoreElements=oTilt.oMot_.oState_.oFilterDataForSpeedControlIqRef_.afConstantsB_.h2  IndexOptions=Index vector (dialog)  Indices=1  OutputSizes=1
  Data Store Write4 : DataStoreWrite  DataStoreName=oTilt  DataStoreElements=oTilt.oMot_.oState_.oFilterDataForSpeedControlIqRef_.afConstantsB_.h1  IndexOptions=Index vector (dialog)  Indices=1  OutputSizes=1
  Data Store Write5 : DataStoreWrite  DataStoreName=oTilt  DataStoreElements=oTilt.oMot_.oState_.oFilterDataForSpeedControlIqRef_.afConstantsB_.h0  IndexOptions=Index vector (dialog)  Indices=1  OutputSizes=1
  Data Store Write6 : DataStoreWrite  DataStoreName=oTilt  DataStoreElements=oTilt.oMot_.oState_.oFilterDataForSpeedControlIqRef_.afPreviousInputs_.h0  IndexOptions=Index vector (dialog)  Indices=1  OutputSizes=1
  Data Store Write7 : DataStoreWrite  DataStoreName=oTilt  DataStoreElements=oTilt.oMot_.oState_.oFilterDataForSpeedControlIqRef_.afPreviousInputs_.h1  IndexOptions=Index vector (dialog)  Indices=1  OutputSizes=1
  Data Store Write8 : DataStoreWrite  DataStoreName=oTilt  DataStoreElements=oTilt.oMot_.oState_.oFilterDataForSpeedControlIqRef_.afPreviousOutputs_.h0  IndexOptions=Index vector (dialog)  Indices=1  OutputSizes=1
  Data Store Write9 : DataStoreWrite  DataStoreName=oTilt  DataStoreElements=oTilt.oMot_.oState_.oFilterDataForSpeedControlIqRef_.afPreviousOutputs_.h1  IndexOptions=Index vector (dialog)  Indices=1  OutputSizes=1
  Data Type Conversion{1..5} (5 alike) : DataTypeConversion  OutDataTypeStr=single
  Demux : Demux  Outputs=6
  Divide : Product  Inputs=*/  OutDataTypeStr=single
  computeCoefficientsButter() : Subsystem
  fActualFrequencyHz : Outport
  wires:
  Data Type Conversion5/1 -> Data Store Write2/1
  Data Type Conversion4/1 -> Data Store Write1/1
  Data Type Conversion3/1 -> Data Store Write3/1
  Data Type Conversion2/1 -> Data Store Write4/1
  Data Type Conversion1/1 -> Data Store Write5/1
  fFreqSample/1 -> computeCoefficientsButter()/2(dSampleFrequencyHz)
  Constant1/1 -> Data Store Write6/1, Data Store Write7/1, Data Store Write9/1, Data Store Write10/1, Data Store Write8/1
  Demux/1 -> Data Type Conversion1/1
  Demux/2 -> Data Type Conversion2/1
  Constant/1 -> Divide/1
  Divide/1 -> Data Store Write/1
  Demux/4 -> Divide/2
  Demux/3 -> Data Type Conversion3/1
  Demux/5 -> Data Type Conversion4/1
  Demux/6 -> Data Type Conversion5/1
  computeCoefficientsButter()/1(dpOutArray) -> Demux/1
  fFreq3db/1 -> computeCoefficientsButter()/1(fCutoffFrequencyHz)
  computeCoefficientsButter()/2(fFreq3db) -> fActualFrequencyHz/1

== system Target_Control_System/Target_Control_System/Simulation Controls/Simulation Data Store Initialization/setupPwm(&oTilt)/setPwmFrequencyApplication()_tilt/setPwmFrequency()_tilt/updateObserver()_tilt ==
  oIsr_.oParam_.fControlLoopDt_ : Inport
  fObserverLoopFilterBandwidthHz_ : Inport  Port=2
  Constant : Constant  Value=15*2*pi  OutDataTypeStr=single
  Constant1 : Constant  Value=8*2*pi  OutDataTypeStr=single
  Constant2 : Constant  Value=2*pi  OutDataTypeStr=single
  Constant3 : Constant  Value=500  OutDataTypeStr=single
  Constant4 : Constant  Value=20  OutDataTypeStr=single
  Constant5 : Constant  Value=100*2*pi  OutDataTypeStr=single
  Constant6 : Constant  Value=4*2*pi  OutDataTypeStr=single
  Constant7 : Constant  Value=0.0625  OutDataTypeStr=single
  Data Store Write : DataStoreWrite  DataStoreName=oTilt  DataStoreElements=oTilt.oIsr_.oParam_.fALpf4hpfDcBlocking_  IndexOptions=Index vector (dialog)  Indices=1  OutputSizes=1
  Data Store Write1 : DataStoreWrite  DataStoreName=oTilt  DataStoreElements=oTilt.oIsr_.oParam_.fAFluxMagnitude_  IndexOptions=Index vector (dialog)  Indices=1  OutputSizes=1
  Data Store Write2 : DataStoreWrite  DataStoreName=oTilt  DataStoreElements=oTilt.oIsr_.oParam_.fALoopfilter2_  IndexOptions=Index vector (dialog)  Indices=1  OutputSizes=1
  Data Store Write3 : DataStoreWrite  DataStoreName=oTilt  DataStoreElements=oTilt.oMot_.oParam_.fObserverLoopFilterBandwidthHz_  IndexOptions=Index vector (dialog)  Indices=1  OutputSizes=1
  Data Store Write4 : DataStoreWrite  DataStoreName=oTilt  DataStoreElements=oTilt.oIsr_.oParam_.fAOmegaFilter2_  IndexOptions=Index vector (dialog)  Indices=1  OutputSizes=1
  Data Store Write5 : DataStoreWrite  DataStoreName=oTilt  DataStoreElements=oTilt.oMot_.oParam_.fAOmegaXfilter2_  IndexOptions=Index vector (dialog)  Indices=1  OutputSizes=1
  Data Store Write6 : DataStoreWrite  DataStoreName=oTilt  DataStoreElements=oTilt.oIsr_.oParam_.oPiDataPll2_.oParameter_.fKp_  IndexOptions=Index vector (dialog)  Indices=1  OutputSizes=1
  Divide{,1,3..4} (4 alike) : Product  Inputs=**
  Divide2 : Product  Inputs=***
  Divide5 : Product  Inputs=*/
  GreaterThan : RelationalOperator  Operator=<  OutDataTypeStr=boolean  RndMeth=Simplest
  Saturation{,1..4} (5 alike) : Saturate  UpperLimit=1.0  LowerLimit=1e-6
  Switch : Switch  Criteria=u2 > Threshold
  wires:
  Divide5/1 -> Data Store Write6/1
  Constant7/1 -> Divide5/1
  Saturation4/1 -> Data Store Write5/1
  oIsr_.oParam_.fControlLoopDt_/1 -> Divide/1, Divide1/1, Divide3/1, Divide2/2, Divide5/2, Divide4/1
  Divide4/1 -> Saturation4/1
  Constant6/1 -> Divide4/2
  Saturation3/1 -> Data Store Write4/1
  Divide3/1 -> Saturation3/1
  Constant5/1 -> Divide3/2
  Switch/1 -> Data Store Write3/1, Divide2/1
  Constant3/1 -> Switch/1
  GreaterThan/1 -> Switch/2
  Constant4/1 -> GreaterThan/2
  fObserverLoopFilterBandwidthHz_/1 -> Switch/3, GreaterThan/1
  Divide2/1 -> Saturation2/1
  Saturation2/1 -> Data Store Write2/1
  Constant2/1 -> Divide2/3
  Divide1/1 -> Saturation1/1
  Saturation1/1 -> Data Store Write1/1
  Constant1/1 -> Divide1/2
  Saturation/1 -> Data Store Write/1
  Divide/1 -> Saturation/1
  Constant/1 -> Divide/2

== system Target_Control_System/Target_Control_System/Simulation Controls/Simulation Data Store Initialization/setupPwm(&oTilt)/setPwmFrequencyApplication()_tilt/setPwmFrequency()_tilt/updateServoObserver()_tilt ==
  oIsr_.oParam_.fControlLoopDt_ : Inport  OutDataTypeStr=double
  fOmegaEDifferentiatorBandwidthHz_ : Inport  Port=2
  Constant : Constant  OutDataTypeStr=single
  Data Store Write : DataStoreWrite  DataStoreName=oTilt  DataStoreElements=oTilt.oMot_.oState_.oPosSensor_.fOmegaEDifferentiatorBandwidthHz_  IndexOptions=Index vector (dialog)  Indices=1  OutputSizes=1
  Divide : Product  Inputs=*/  OutDataTypeStr=single
  softwareIirFilterInitialize() : Subsystem  TreatAsAtomicUnit=on
  wires:
  fOmegaEDifferentiatorBandwidthHz_/1 -> softwareIirFilterInitialize()/1(fFreq3db)
  Divide/1 -> softwareIirFilterInitialize()/2(fFreqSample)
  oIsr_.oParam_.fControlLoopDt_/1 -> Divide/2
  softwareIirFilterInitialize()/1(fActualFrequencyHz) -> Data Store Write/1
  Constant/1 -> Divide/1

== system Target_Control_System/Target_Control_System/Simulation Controls/Simulation Data Store Initialization/setupPwm()/setPwmFrequencyApplication()_pitch/setPwmFrequency()_pitch/softwareIirFilterInitialize() ==
  fFreq3db : Inport
  fFreqSample : Inport  Port=2
  Constant : Constant  OutDataTypeStr=single
  Constant1 : Constant  Value=0  OutDataTypeStr=single
  Data Store Write : DataStoreWrite  DataStoreName=oPitch  DataStoreElements=oPitch.oMot_.oState_.oMotorAccelerationFilterStage1_.afConstantsA_.h0  IndexOptions=Index vector (dialog)  Indices=1  OutputSizes=1
  Data Store Write1 : DataStoreWrite  DataStoreName=oPitch  DataStoreElements=oPitch.oMot_.oState_.oMotorAccelerationFilterStage1_.afConstantsA_.h1  IndexOptions=Index vector (dialog)  Indices=1  OutputSizes=1
  Data Store Write10 : DataStoreWrite  DataStoreName=oPitch  DataStoreElements=oPitch.oMot_.oState_.oMotorAccelerationFilterStage1_.fFilterOutput_  IndexOptions=Index vector (dialog)  Indices=1  OutputSizes=1
  Data Store Write2 : DataStoreWrite  DataStoreName=oPitch  DataStoreElements=oPitch.oMot_.oState_.oMotorAccelerationFilterStage1_.afConstantsA_.h2  IndexOptions=Index vector (dialog)  Indices=1  OutputSizes=1
  Data Store Write3 : DataStoreWrite  DataStoreName=oPitch  DataStoreElements=oPitch.oMot_.oState_.oMotorAccelerationFilterStage1_.afConstantsB_.h2  IndexOptions=Index vector (dialog)  Indices=1  OutputSizes=1
  Data Store Write4 : DataStoreWrite  DataStoreName=oPitch  DataStoreElements=oPitch.oMot_.oState_.oMotorAccelerationFilterStage1_.afConstantsB_.h1  IndexOptions=Index vector (dialog)  Indices=1  OutputSizes=1
  Data Store Write5 : DataStoreWrite  DataStoreName=oPitch  DataStoreElements=oPitch.oMot_.oState_.oMotorAccelerationFilterStage1_.afConstantsB_.h0  IndexOptions=Index vector (dialog)  Indices=1  OutputSizes=1
  Data Store Write6 : DataStoreWrite  DataStoreName=oPitch  DataStoreElements=oPitch.oMot_.oState_.oMotorAccelerationFilterStage1_.afPreviousInputs_.h0  IndexOptions=Index vector (dialog)  Indices=1  OutputSizes=1
  Data Store Write7 : DataStoreWrite  DataStoreName=oPitch  DataStoreElements=oPitch.oMot_.oState_.oMotorAccelerationFilterStage1_.afPreviousInputs_.h1  IndexOptions=Index vector (dialog)  Indices=1  OutputSizes=1
  Data Store Write8 : DataStoreWrite  DataStoreName=oPitch  DataStoreElements=oPitch.oMot_.oState_.oMotorAccelerationFilterStage1_.afPreviousOutputs_.h0  IndexOptions=Index vector (dialog)  Indices=1  OutputSizes=1
  Data Store Write9 : DataStoreWrite  DataStoreName=oPitch  DataStoreElements=oPitch.oMot_.oState_.oMotorAccelerationFilterStage1_.afPreviousOutputs_.h1  IndexOptions=Index vector (dialog)  Indices=1  OutputSizes=1
  Data Type Conversion{1..5} (5 alike) : DataTypeConversion  OutDataTypeStr=single
  Demux : Demux  Outputs=6
  Divide : Product  Inputs=*/  OutDataTypeStr=single
  computeCoefficientsButter() : Subsystem
  fActualFrequencyHz : Outport
  wires:
  Data Type Conversion5/1 -> Data Store Write2/1
  Data Type Conversion4/1 -> Data Store Write1/1
  Data Type Conversion3/1 -> Data Store Write3/1
  Data Type Conversion1/1 -> Data Store Write4/1
  Data Type Conversion2/1 -> Data Store Write5/1
  fFreqSample/1 -> computeCoefficientsButter()/2(dSampleFrequencyHz)
  Constant1/1 -> Data Store Write6/1, Data Store Write7/1, Data Store Write9/1, Data Store Write10/1, Data Store Write8/1
  Demux/1 -> Data Type Conversion2/1
  Demux/2 -> Data Type Conversion1/1
  Constant/1 -> Divide/1
  Divide/1 -> Data Store Write/1
  Demux/4 -> Divide/2
  Demux/3 -> Data Type Conversion3/1
  Demux/5 -> Data Type Conversion4/1
  Demux/6 -> Data Type Conversion5/1
  computeCoefficientsButter()/1(dpOutArray) -> Demux/1
  fFreq3db/1 -> computeCoefficientsButter()/1(fCutoffFrequencyHz)
  computeCoefficientsButter()/2(fFreq3db) -> fActualFrequencyHz/1
